simulink model "untitled"  (R2019a)
settings: Solver=VariableStepAuto  StartTime=0.0  StopTime=10.0  RelTol=1e-3
settings Model: Creator=mengc  LastModifiedBy=mengc

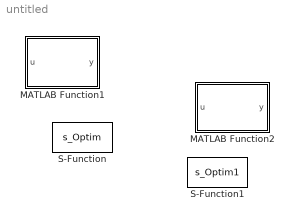
== system untitled ==
  MATLAB Function1 : MATLAB Function  TreatAsAtomicUnit=on
  MATLAB Function2 : MATLAB Function  TreatAsAtomicUnit=on
  S-Function : S-Function  FunctionName=s_Optim  SFunctionDeploymentMode=off  EnableBusSupport=off
  S-Function1 : S-Function  FunctionName=s_Optim1  SFunctionDeploymentMode=off  EnableBusSupport=off

== matlab function untitled/MATLAB Function1 ==
  data: u input; y output
function y = optim(u)
K=1*[-0.56   0       0.56    0;
          0  -0.56    0       0.56;
      0.218   0.218   0.218   0.218];
a=0.3490000;
e=u;
e=e/norm(e);
cf = @(x)confun(x,e,K);
of = @(x)objfun(x,K);
% A=[];b=[];Aeq=[];beq=[];
A=-e'*K;b=0;Aeq=[0 -e(3) e(2);e(3) 0 -e(1);-e(2) e(1) 0]*K;beq=[0;0;0];
lb=[-a,-a,-a,-a];ub=[a,a,a,a];
options = optimoptions(@ fmincon,'Algorithm','interior-point','Display','iter');
% x0=[0;0;0;0]; %对解决方案进行初步猜测
c1=-e(1)+0.5*e(3);c2=-e(2)+0.5*e(3);c3= e(1)+0.5*e(3);c4= e(2)+0.5*e(3);
x0=0.05*[c1;c2;c3;c4];
x = fmincon(of,x0,A,b,Aeq,beq,lb,ub,[],options);
U=K*x;

if(normest(u)>=normest(U))
    y = x;
else
    y = Torque2surface1(u);
end

== matlab function untitled/MATLAB Function2 ==
  data: u input; y output
function y = Torque2surface1(u)
% 无舵面调整
%---------限幅---------
u(1)=Constrain(u(1),-0.39088,0.39088);
u(2)=Constrain(u(2),-0.39088,0.39088);
u(3)=Constrain(u(3),-0.3043,0.3043);
%----------------------
k=[-0.8929         0    1.1468;
         0   -0.8929    1.1468;
    0.8929         0    1.1468;
         0    0.8929    1.1468];
y = k*u;
